simulink model "Simple_4Quad_payload_01"  (R2018b)
settings: Solver=VariableStepAuto  StartTime=0.0  StopTime=60  RelTol=1e-3
InitFcn:
  | Simple_4Quad_payload_01_const
values from neighbouring files (symbols this model uses):
  d1 = 0.25    [Colab_4Quad_model_01_const.m]    (also in Colab_4Quad_model_02_const.m = 0.5; Simple_4Quad_payload_01_const.m = 1; Simple_4Quad_payload_02_const.m = 1; Simple_4Quad_payload_03_const.m = 1)
  d2 = 0.25    [Colab_4Quad_model_01_const.m]    (also in Colab_4Quad_model_02_const.m = 0.5; Simple_4Quad_payload_01_const.m = 1; Simple_4Quad_payload_02_const.m = 1; Simple_4Quad_payload_03_const.m = 1)
  Des_rel_dist = 2    [Simple_4Quad_payload_01_const.m]    (also in Simple_4Quad_payload_02_const.m = 4; Simple_4Quad_payload_03_const.m = 4; Simple_4Quad_payload_04_const.m; Simple_4Quad_payload_05_const.m)
  g = 9.81    [Colab_4Quad_model_01_const.m]    (also in Colab_4Quad_model_02_const.m; Simple_2Quad_payload_01_const.m; Simple_2Quad_payload_02_const.m; Simple_2Quad_payload_03_const.m)
  Ix = 0.166667    [Colab_4Quad_model_01_const.m]    (also in Colab_4Quad_model_02_const.m = 0.02; Simple_4Quad_payload_01_const.m = 1; Simple_4Quad_payload_02_const.m = 1; Simple_4Quad_payload_03_const.m = 1)
  Iy = 0.166667    [Colab_4Quad_model_01_const.m]    (also in Colab_4Quad_model_02_const.m = 0.02; Simple_4Quad_payload_01_const.m = 1; Simple_4Quad_payload_02_const.m = 1; Simple_4Quad_payload_03_const.m = 1)
  Iz = 0.166667    [Colab_4Quad_model_01_const.m]    (also in Colab_4Quad_model_02_const.m = 0.02; Simple_4Quad_payload_01_const.m = 1; Simple_4Quad_payload_02_const.m = 1; Simple_4Quad_payload_03_const.m = 1)
  l = 3.1819    [Colab_4Quad_model_01_const.m]    (also in Colab_4Quad_model_02_const.m = 3; Simple_2Quad_payload_04_const.m = 1; Simple_4Quad_payload_01_const.m = 1; Simple_4Quad_payload_02_const.m = 2)
  m = 1.5    [Colab_4Quad_model_01_const.m]    (also in Colab_4Quad_model_02_const.m; Simple_2Quad_payload_04_const.m = 1; Simple_4Quad_payload_01_const.m = 1; Simple_4Quad_payload_02_const.m = 1)
  M = 1.0    (= 1)    [Colab_4Quad_model_01_const.m]    (also in Colab_4Quad_model_02_const.m; Simple_2Quad_payload_01_const.m; Simple_2Quad_payload_02_const.m; Simple_2Quad_payload_03_const.m)
  Md = 1*[1;1;1]    [Simple_2Quad_payload_04_const.m]    (also in Simple_4Quad_payload_01_const.m = 1*[1;1;1;1;1;1]; Simple_4Quad_payload_02_const.m = 1*[1;1;1;1;1;1]; Simple_4Quad_payload_03_const.m = 1*[1;1;1;1;1;1]; Simple_4Quad_payload_04_const.m = 1*[1;1;1;1;1;1])
libraries: simulink x16
(part 2 of 2)

== system Simple_4Quad_payload_01/Agent4/PID_beta4 ==
  beta4_des : Inport
  beta4 : Inport  Port=2
  D_beta4 : Inport  Port=3
  PID Controller : simulink/Continuous/PID Controller  Controller=PID  Form=Parallel  TimeDomain=Continuous-time  SampleTime=-1  IntegratorMethod=Forward Euler  FilterMethod=Forward Euler  ControllerParametersSource=internal  P=10  I=1  D=0  UseFilter=on  N=100  TunerSelectOption=Transfer Function Based (PID Tuner App)  InitialConditionSource=internal  InitialConditionForIntegrator=0  InitialConditionForFilter=0  DifferentiatorICPrevScaledInput=0  ExternalReset=none  TrackingMode=off  Kt=1  LimitOutput=off  UpperSaturationLimit=inf  LowerSaturationLimit=-inf  LinearizeAsGain=on  AntiWindupMode=none  Kb=1  POutMin=[]  POutMax=[]  IOutMin=[]  IOutMax=[]  DOutMin=[]  DOutMax=[]  NOutMin=[]  NOutMax=[]  SumOutMin=[]  SumOutMax=[]  SaturationOutMin=[]  SaturationOutMax=[]  PParamMin=[]  PParamMax=[]  IParamMin=[]  IParamMax=[]  DParamMin=[]  DParamMax=[]  NParamMin=[]  NParamMax=[]  KbParamMin=[]  KbParamMax=[]  KtParamMin=[]  KtParamMax=[]  KbOutMin=[]  KbOutMax=[]  KtOutMin=[]  KtOutMax=[]  IntegratorOutMin=[]  IntegratorOutMax=[]  FilterOutMin=[]  FilterOutMax=[]  SumI1OutMin=[]  SumI1OutMax=[]  SumI2OutMin=[]  SumI2OutMax=[]  SumI3OutMin=[]  SumI3OutMax=[]  SumI4OutMin=[]  SumI4OutMax=[]  SumDOutMin=[]  SumDOutMax=[]  DifferentiatorOutMin=[]  DifferentiatorOutMax=[]  FilterDiffOutCoefMin=[]  FilterDiffOutCoefMax=[]  ReciprocalOutMin=[]  ReciprocalOutMax=[]  SumDenOutMin=[]  SumDenOutMax=[]  SumNumOutMin=[]  SumNumOutMax=[]  DivideOutMin=[]  DivideOutMax=[]  IntegratorContinuousStateAttributes=''  IntegratorStateMustResolveToSignalObject=off  IntegratorRTWStateStorageClass=Auto  FilterContinuousStateAttributes=''  FilterStateMustResolveToSignalObject=off  FilterRTWStateStorageClass=Auto  ParallelPVariant=InternalParameters  IdealPVariant=Disabled  IVariant=InternalParameters  DVariant=InternalParameters  IntegratorVariant=Continuous  SatVariant=Disabled  AWVariant=Passthrough  PCopyVariant=Disabled  TRVariant=Disabled  FdbkBlocksVariant=Forward  IdealPFdbkVariant=Disabled  SatFdbkVariant=Disabled  DerivativeFilterVariant=ContFilter  NVariant=InternalParameters  NCopyVariant=Disabled  FilterICVariant=InternalICsFilter  IntegratorICVariant=InternalICs  ExternalResetVariant=Disabled  TRSumVariant=Passthrough  SumFdbkVariant=Disabled  SumVariant=Sum_PID
  PID Controller1 : simulink/Continuous/PID Controller  Controller=PID  Form=Parallel  TimeDomain=Continuous-time  SampleTime=-1  IntegratorMethod=Forward Euler  FilterMethod=Forward Euler  ControllerParametersSource=internal  P=100  I=0  D=0  UseFilter=on  N=100  TunerSelectOption=Transfer Function Based (PID Tuner App)  InitialConditionSource=internal  InitialConditionForIntegrator=0  InitialConditionForFilter=0  DifferentiatorICPrevScaledInput=0  ExternalReset=none  TrackingMode=off  Kt=1  LimitOutput=off  UpperSaturationLimit=inf  LowerSaturationLimit=-inf  LinearizeAsGain=on  AntiWindupMode=none  Kb=1  POutMin=[]  POutMax=[]  IOutMin=[]  IOutMax=[]  DOutMin=[]  DOutMax=[]  NOutMin=[]  NOutMax=[]  SumOutMin=[]  SumOutMax=[]  SaturationOutMin=[]  SaturationOutMax=[]  PParamMin=[]  PParamMax=[]  IParamMin=[]  IParamMax=[]  DParamMin=[]  DParamMax=[]  NParamMin=[]  NParamMax=[]  KbParamMin=[]  KbParamMax=[]  KtParamMin=[]  KtParamMax=[]  KbOutMin=[]  KbOutMax=[]  KtOutMin=[]  KtOutMax=[]  IntegratorOutMin=[]  IntegratorOutMax=[]  FilterOutMin=[]  FilterOutMax=[]  SumI1OutMin=[]  SumI1OutMax=[]  SumI2OutMin=[]  SumI2OutMax=[]  SumI3OutMin=[]  SumI3OutMax=[]  SumI4OutMin=[]  SumI4OutMax=[]  SumDOutMin=[]  SumDOutMax=[]  DifferentiatorOutMin=[]  DifferentiatorOutMax=[]  FilterDiffOutCoefMin=[]  FilterDiffOutCoefMax=[]  ReciprocalOutMin=[]  ReciprocalOutMax=[]  SumDenOutMin=[]  SumDenOutMax=[]  SumNumOutMin=[]  SumNumOutMax=[]  DivideOutMin=[]  DivideOutMax=[]  IntegratorContinuousStateAttributes=''  IntegratorStateMustResolveToSignalObject=off  IntegratorRTWStateStorageClass=Auto  FilterContinuousStateAttributes=''  FilterStateMustResolveToSignalObject=off  FilterRTWStateStorageClass=Auto  ParallelPVariant=InternalParameters  IdealPVariant=Disabled  IVariant=InternalParameters  DVariant=InternalParameters  IntegratorVariant=Continuous  SatVariant=Disabled  AWVariant=Passthrough  PCopyVariant=Disabled  TRVariant=Disabled  FdbkBlocksVariant=Forward  IdealPFdbkVariant=Disabled  SatFdbkVariant=Disabled  DerivativeFilterVariant=ContFilter  NVariant=InternalParameters  NCopyVariant=Disabled  FilterICVariant=InternalICsFilter  IntegratorICVariant=InternalICs  ExternalResetVariant=Disabled  TRSumVariant=Passthrough  SumFdbkVariant=Disabled  SumVariant=Sum_PID
  Scope3 : Scope  NumInputPorts=3
  Sum : Sum  Inputs=|+-
  Sum1 : Sum  Inputs=|+-
  S4 : Outport
  wires:
  D_beta4/1 -> Sum1/2
  PID Controller/1 -> Sum1/1
  PID Controller1/1 -> S4/1, Scope3/3
  Sum/1 -> Scope3/1, PID Controller/1
  Sum1/1 -> PID Controller1/1, Scope3/2
  beta4_des/1 -> Sum/1
  beta4/1 -> Sum/2

== matlab function Simple_4Quad_payload_01/payload/Controller ==
  data: e input; F output; alphas_des output; PHI input; alphas input; betas input; betas_des output; Md parameter; g parameter; M parameter; OUT output; d1 parameter; d2 parameter; Ix parameter; Iy parameter; Iz parameter; l parameter; Des_rel_dist parameter; B output; U output
function [F,alphas_des,betas_des,OUT,B,U] = fcn(e,PHI,alphas,betas, Md, g, M, d1, d2, Ix, Iy, Iz, l, Des_rel_dist)

phi = PHI(1);
theta = PHI(2);
psi = PHI(3);

alpha1 = alphas(1);
alpha2 = alphas(2);
alpha3 = alphas(3);
alpha4 = alphas(4);

beta1 = betas(1);
beta2 = betas(2);
beta3 = betas(3);
beta4 = betas(4);

Io = diag([Ix;Iy;Iz]);

Ro = [cos(psi)*cos(theta) cos(psi)*sin(theta)*sin(phi)-sin(psi)*cos(phi) cos(psi)*sin(theta)*cos(phi)+sin(psi)*sin(phi);
    sin(psi)*cos(theta) sin(psi)*sin(theta)*sin(phi)+cos(psi)*cos(phi) sin(psi)*sin(theta)*cos(phi)-cos(psi)*sin(phi);
    -sin(theta) cos(theta)*sin(phi) cos(theta)*cos(phi)];

A = [Io^(-1) zeros(3);
    zeros(3) (1/M)*Ro];

B1 = [0 0 d2*(sin(alpha3)) -d2*(sin(alpha4));
    -d1*(sin(alpha1)) d1*(sin(alpha2)) 0 0;
    d1*cos(alpha1)*sin(beta1) -d1*cos(alpha2)*sin(beta2) d2*cos(alpha3)*sin(beta3) -d2*cos(alpha4)*sin(beta4)];

B2 = [cos(alpha1)*cos(beta1) cos(alpha2)*cos(beta2) -cos(alpha3)*sin(beta3) -cos(alpha4)*sin(beta4);
    cos(alpha1)*sin(beta1) cos(alpha2)*sin(beta2) cos(alpha3)*cos(beta3) cos(alpha4)*cos(beta4);
    sin(alpha1) sin(alpha2) sin(alpha3) sin(alpha4)];

B = [B1;B2];

D = [0;0;0;0;0;-g];

SGN = zeros(6);
for i=1:6
    SGN(i,i) = e(i)/(abs(e(i))+0.1);
end

Z = SGN*Md;
U = Z - D;
F = ((B'*(A'*A)*B)^(-1))*(B'*A')*U; %1*g/4*[1;1;1;1];

beta1_des = asin(2*tan(alpha1)*U(5)/U(6));
beta2_des = pi - asin(2*tan(alpha2)*U(5)/U(6));
beta3_des = asin(-2*tan(alpha3)*U(4)/U(6));
beta4_des = pi - asin(-2*tan(alpha4)*U(4)/U(6));

alpha1_des = acos( (Des_rel_dist/2 - d1)/l );
alpha2_des = acos( (Des_rel_dist/2 - d1)/l );
alpha3_des = acos( (Des_rel_dist/2 - d2)/l );
alpha4_des = acos( (Des_rel_dist/2 - d2)/l );

betas_des = [beta1_des;beta2_des;beta3_des;beta4_des];
alphas_des = [alpha1_des;alpha2_des;alpha3_des;alpha4_des];

OUT = U;

end

== matlab function Simple_4Quad_payload_01/payload/Dynamic Model ==
  data: fs input; DD_PHI output; alphas input; betas input; PHI input; DD_P output; d2 parameter; M parameter; Ix parameter; g parameter; Iy parameter; Iz parameter; d1 parameter; R1 output; R2 output; R3 output; R4 output; Ro output
function [DD_PHI,DD_P,R1,R2,R3,R4,Ro] = fcn(fs,alphas,betas,PHI,d2, M, Ix,g, Iy, Iz, d1)

f1 = fs(1);
f2 = fs(2);
f3 = fs(3);
f4 = fs(4);

alpha1 = alphas(1);
alpha2 = alphas(2);
alpha3 = alphas(3);
alpha4 = alphas(4);

beta1 = betas(1);
beta2 = betas(2);
beta3 = betas(3);
beta4 = betas(4);

phi = PHI(1);
theta = PHI(2);
psi = PHI(3);

Io = diag([Ix;Iy;Iz]);

R1 = [cos(alpha1)*cos(beta1) -sin(beta1) -sin(alpha1)*cos(beta1);
    cos(alpha1)*sin(beta1) cos(beta1) -sin(alpha1)*sin(beta1);
    sin(alpha1) 0 cos(alpha1)];

R2 = [cos(alpha2)*cos(beta2) -sin(beta2) -sin(alpha2)*cos(beta2);
    cos(alpha2)*sin(beta2) cos(beta2) -sin(alpha2)*sin(beta2);
    sin(alpha2) 0 cos(alpha2)];

R3 = [cos(alpha3)*cos(beta3) -sin(beta3) -sin(alpha3)*cos(beta3);
    cos(alpha3)*sin(beta3) cos(beta3) -sin(alpha3)*sin(beta3);
    sin(alpha3) 0 cos(alpha3)];

R4 = [cos(alpha4)*cos(beta4) -sin(beta4) -sin(alpha4)*cos(beta4);
    cos(alpha4)*sin(beta4) cos(beta4) -sin(alpha4)*sin(beta4);
    sin(alpha4) 0 cos(alpha4)];

Ro = [cos(psi)*cos(theta) cos(psi)*sin(theta)*sin(phi)-sin(psi)*cos(phi) cos(psi)*sin(theta)*cos(phi)+sin(psi)*sin(phi);
    sin(psi)*cos(theta) sin(psi)*sin(theta)*sin(phi)+cos(psi)*cos(phi) sin(psi)*sin(theta)*cos(phi)-cos(psi)*sin(phi);
    -sin(theta) cos(theta)*sin(phi) cos(theta)*cos(phi)];

F1 = [f1;0;0];
F2 = [f2;0;0];
F3 = [f3;0;0];
F4 = [f4;0;0];

r1 = [d1;0;0];
r2 = [-d1;0;0];
r3 = [0;d2;0];
r4 = [0;-d2;0];

G = [0;0;-g];

DD_PHI = (Io^(-1)) * ( External_Product3(r1,F1) + External_Product3(r2,F2) + External_Product3(r3,F3) + External_Product3(r4,F4) );
DD_P = (1/M) * ( ( Ro * ( R1*F1 + R2*F2 + R3*F3 + R4*F4 ) ) + M*G );

end

== matlab function Simple_4Quad_payload_01/Agent2/Dynamic Model2 ==
  data: DD_alpha2 output; N2 input; S2 input; f2 input; alpha2 input; beta2 input; D_alpha2 input; D_beta2 input; m parameter; g parameter; DD_PHI input; DD_P input; D_PHI input; l parameter; d1 parameter; PHI input; DD_beta2 output; U2 output; P input; P2 output
function [DD_alpha2,DD_beta2,U2,P2]  = fcn(N2,S2,f2,alpha2,beta2,D_alpha2,D_beta2,m, g,DD_PHI,DD_P,D_PHI, l, d1,PHI,P)

phi = PHI(1);
theta = PHI(2);
psi = PHI(3);

Dist2_local = [-d1;0;0];
D2_angles = [0;D_alpha2;D_beta2];

Ro = [cos(psi)*cos(theta) cos(psi)*sin(theta)*sin(phi)-sin(psi)*cos(phi) cos(psi)*sin(theta)*cos(phi)+sin(psi)*sin(phi);
    sin(psi)*cos(theta) sin(psi)*sin(theta)*sin(phi)+cos(psi)*cos(phi) sin(psi)*sin(theta)*cos(phi)-cos(psi)*sin(phi);
    -sin(theta) cos(theta)*sin(phi) cos(theta)*cos(phi)];

R2 = [cos(alpha2)*cos(beta2) -sin(beta2) sin(alpha2)*cos(beta2);
    cos(alpha2)*sin(beta2) cos(beta2) sin(alpha2)*sin(beta2);
    -sin(alpha2) 0 cos(alpha2)];

C1_2 = External_Product3(D_PHI,Dist2_local);
C2_2 = External_Product3(D_PHI,C1_2);
C3_2 = External_Product3(DD_PHI,Dist2_local);

C4_2 = External_Product3(D2_angles,Dist2_local);
C5_2 = External_Product3(D2_angles,C4_2);

a2_part = (  R2' * ( Ro'*DD_P + C2_2 + C3_2 ) ) + C5_2;

G2_local = R2' * Ro' * [0;0;-g];

T2 = m*a2_part(1) + f2 - m*G2_local(1);
DD_alpha2 = (1/m/l) * (N2 - m*a2_part(2) + m*G2_local(2));
DD_beta2 = (1/m/l) * (S2 - m*a2_part(3) + m*G2_local(3));

U2 = R2 * [T2;N2;S2];

P2 = P + Ro*Dist2_local + Ro*R2*[l;0;0];

end

== matlab function Simple_4Quad_payload_01/Agent1 /Dynamic Model1 ==
  data: DD_alpha1 output; N1 input; S1 input; f1 input; alpha1 input; beta1 input; D_alpha1 input; D_beta1 input; m parameter; g parameter; DD_PHI input; DD_P input; D_PHI input; l parameter; d1 parameter; PHI input; DD_beta1 output; U1 output; P input; P1 output
function [DD_alpha1,DD_beta1,U1,P1]  = fcn(N1,S1,f1,alpha1,beta1,D_alpha1,D_beta1,m, g,DD_PHI,DD_P,D_PHI, l, d1,PHI,P)

phi = PHI(1);
theta = PHI(2);
psi = PHI(3);

Dist1_local = [d1;0;0];
D1_angles = [0;D_alpha1;D_beta1];

Ro = [cos(psi)*cos(theta) cos(psi)*sin(theta)*sin(phi)-sin(psi)*cos(phi) cos(psi)*sin(theta)*cos(phi)+sin(psi)*sin(phi);
    sin(psi)*cos(theta) sin(psi)*sin(theta)*sin(phi)+cos(psi)*cos(phi) sin(psi)*sin(theta)*cos(phi)-cos(psi)*sin(phi);
    -sin(theta) cos(theta)*sin(phi) cos(theta)*cos(phi)];

R1 = [cos(alpha1)*cos(beta1) -sin(beta1) sin(alpha1)*cos(beta1);
    cos(alpha1)*sin(beta1) cos(beta1) sin(alpha1)*sin(beta1);
    -sin(alpha1) 0 cos(alpha1)];

C1_1 = External_Product3(D_PHI,Dist1_local);
C2_1 = External_Product3(D_PHI,C1_1);
C3_1 = External_Product3(DD_PHI,Dist1_local);

C4_1 = External_Product3(D1_angles,Dist1_local);
C5_1 = External_Product3(D1_angles,C4_1);

a1_part = (  R1' * ( Ro'*DD_P + C2_1 + C3_1 ) ) + C5_1;

G1_local = R1' * Ro' * [0;0;-g];

T1 = m*a1_part(1) + f1 - m*G1_local(1);
DD_alpha1 = (1/m/l) * (N1 - m*a1_part(2) + m*G1_local(2));
DD_beta1 = (1/m/l) * (S1 - m*a1_part(3) + m*G1_local(3));

U1 = R1 * [T1;N1;S1];

P1 = P + Ro*Dist1_local + Ro*R1*[l;0;0];

end

== matlab function Simple_4Quad_payload_01/Agent4/Dynamic Model4 ==
  data: DD_alpha4 output; N4 input; S4 input; f4 input; alpha4 input; beta4 input; D_alpha4 input; D_beta4 input; m parameter; g parameter; DD_PHI input; DD_P input; D_PHI input; l parameter; d2 parameter; PHI input; DD_beta4 output; U4 output; P input; P4 output
function [DD_alpha4,DD_beta4,U4,P4]  = fcn(N4,S4,f4,alpha4,beta4,D_alpha4,D_beta4,m, g,DD_PHI,DD_P,D_PHI, l, d2,PHI,P)

phi = PHI(1);
theta = PHI(2);
psi = PHI(3);

Dist4_local = [0;-d2;0];
D4_angles = [0;D_alpha4;D_beta4];

Ro = [cos(psi)*cos(theta) cos(psi)*sin(theta)*sin(phi)-sin(psi)*cos(phi) cos(psi)*sin(theta)*cos(phi)+sin(psi)*sin(phi);
    sin(psi)*cos(theta) sin(psi)*sin(theta)*sin(phi)+cos(psi)*cos(phi) sin(psi)*sin(theta)*cos(phi)-cos(psi)*sin(phi);
    -sin(theta) cos(theta)*sin(phi) cos(theta)*cos(phi)];

R4 = [cos(alpha4)*cos(beta4) -sin(beta4) sin(alpha4)*cos(beta4);
    cos(alpha4)*sin(beta4) cos(beta4) sin(alpha4)*sin(beta4);
    -sin(alpha4) 0 cos(alpha4)];

C1_4 = External_Product3(D_PHI,Dist4_local);
C2_4 = External_Product3(D_PHI,C1_4);
C3_4 = External_Product3(DD_PHI,Dist4_local);

C4_4 = External_Product3(D4_angles,Dist4_local);
C5_4 = External_Product3(D4_angles,C4_4);

a4_part = (  R4' * ( Ro'*DD_P + C2_4 + C3_4 ) ) + C5_4;

G4_local = R4' * Ro' * [0;0;-g];

T4 = m*a4_part(1) + f4 - m*G4_local(1);
DD_alpha4 = (1/m/l) * (N4 - m*a4_part(2) + m*G4_local(2));
DD_beta4 = (1/m/l) * (S4 - m*a4_part(3) + m*G4_local(3));

U4 = R4 * [T4;N4;S4];

P4 = P + Ro*Dist4_local + Ro*R4*[l;0;0];

end

== matlab function Simple_4Quad_payload_01/Agent3/Dynamic Model3 ==
  data: DD_alpha3 output; N3 input; S3 input; f3 input; alpha3 input; beta3 input; D_alpha3 input; D_beta3 input; m parameter; g parameter; DD_PHI input; DD_P input; D_PHI input; l parameter; d2 parameter; PHI input; DD_beta3 output; U3 output; P input; P3 output
function [DD_alpha3,DD_beta3,U3,P3]  = fcn(N3,S3,f3,alpha3,beta3,D_alpha3,D_beta3,m, g,DD_PHI,DD_P,D_PHI, l, d2,PHI,P)

phi = PHI(1);
theta = PHI(2);
psi = PHI(3);

Dist3_local = [0;d2;0];
D3_angles = [0;D_alpha3;D_beta3];

Ro = [cos(psi)*cos(theta) cos(psi)*sin(theta)*sin(phi)-sin(psi)*cos(phi) cos(psi)*sin(theta)*cos(phi)+sin(psi)*sin(phi);
    sin(psi)*cos(theta) sin(psi)*sin(theta)*sin(phi)+cos(psi)*cos(phi) sin(psi)*sin(theta)*cos(phi)-cos(psi)*sin(phi);
    -sin(theta) cos(theta)*sin(phi) cos(theta)*cos(phi)];

R3 = [cos(alpha3)*cos(beta3) -sin(beta3) sin(alpha3)*cos(beta3);
    cos(alpha3)*sin(beta3) cos(beta3) sin(alpha3)*sin(beta3);
    -sin(alpha3) 0 cos(alpha3)];

C1_3 = External_Product3(D_PHI,Dist3_local);
C2_3 = External_Product3(D_PHI,C1_3);
C3_3 = External_Product3(DD_PHI,Dist3_local);

C4_3 = External_Product3(D3_angles,Dist3_local);
C5_3 = External_Product3(D3_angles,C4_3);

a3_part = (  R3' * ( Ro'*DD_P + C2_3 + C3_3 ) ) + C5_3;

G3_local = R3' * Ro' * [0;0;-g];

T3 = m*a3_part(1) + f3 - m*G3_local(1);
DD_alpha3 = (1/m/l) * (N3 - m*a3_part(2) + m*G3_local(2));
DD_beta3 = (1/m/l) * (S3 - m*a3_part(3) + m*G3_local(3));

U3 = R3 * [T3;N3;S3];

P3 = P + Ro*Dist3_local + Ro*R3*[l;0;0];

end
